simulink model "nonlinear_LQG"  (R2021b)
settings: Solver=VariableStepAuto  StartTime=0.0  StopTime=100  RelTol=1e-3
undefined symbols (not defined in the file): C1, K, sysKF
settings Model: Creator=Anubhav Paras  LastModifiedBy=vanshika
settings SolverCC: AlgebraicLoopSolver=TrustRegion
settings DebuggingCC: SFMachineParentedDataDiag=warning

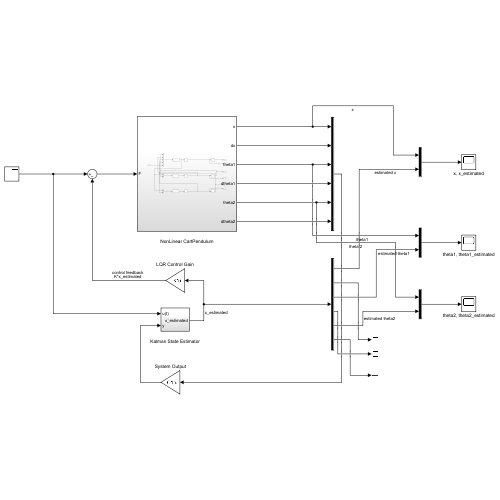
[thumbnail: Simulink's stored preview of the top-level diagram]
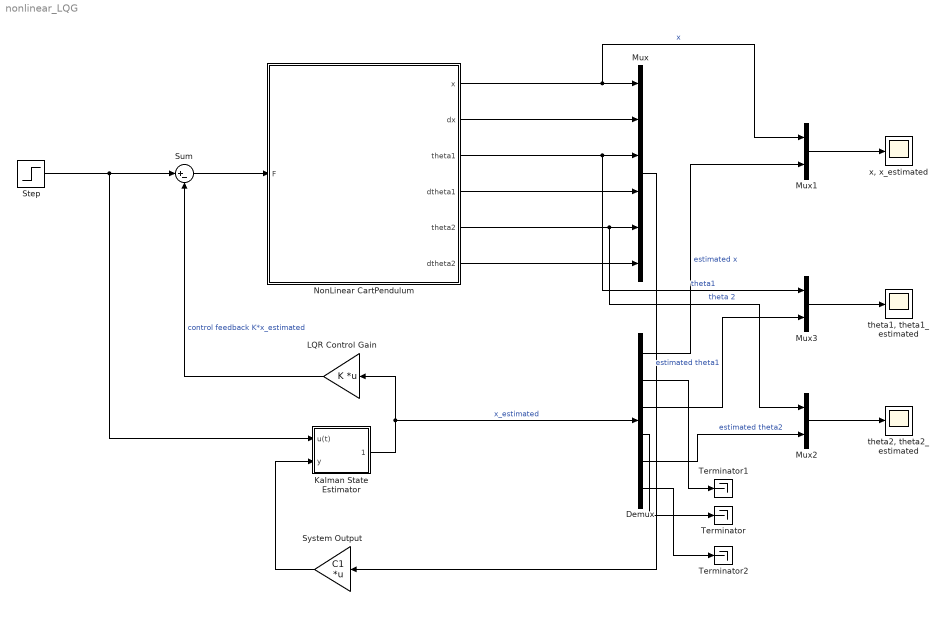
== system nonlinear_LQG ==
  " Kalman State Estimator" : Subsystem
  " NonLinear CartPendulum" : Subsystem
  Demux : Demux  Outputs=6
  LQR Control Gain : Gain  Gain=K  Multiplication=Matrix(K*u)
  Mux : Mux  Inputs=6
  Mux1 : Mux  Inputs=2
  Mux2 : Mux  Inputs=2
  Mux3 : Mux  Inputs=2
  Step : Step  SampleTime=5
  Sum : Sum  Inputs=|+-
  System Output : Gain  Gain=C1  Multiplication=Matrix(K*u)
  Terminator : Terminator
  Terminator1 : Terminator
  Terminator2 : Terminator
  "theta1, theta1_estimated" : Scope
  "theta2, theta2_estimated" : Scope
  "x, x_estimated" : Scope
  wires:
  System Output/1 -> " Kalman State Estimator"/2(y)
  " NonLinear CartPendulum"/1(x) -> Mux1/1, Mux/1  "x"
  Mux3/1 -> "theta1, theta1_estimated"/1
  Demux/1 -> Mux1/2  "estimated x"
  Mux2/1 -> "theta2, theta2_estimated"/1
  " Kalman State Estimator"/1(x_estimated) -> LQR Control Gain/1, Demux/1  "x_estimated"
  Demux/2 -> Terminator1/1
  Demux/4 -> Terminator/1
  Step/1 -> Sum/1, " Kalman State Estimator"/1(u(t))
  " NonLinear CartPendulum"/5(theta2) -> Mux2/1, Mux/5  "theta 2"
  " NonLinear CartPendulum"/2(dx) -> Mux/2
  Demux/5 -> Mux2/2  "estimated theta2"
  Mux1/1 -> "x, x_estimated"/1
  " NonLinear CartPendulum"/6(dtheta2) -> Mux/6
  Mux/1 -> System Output/1
  " NonLinear CartPendulum"/4(dtheta1) -> Mux/4
  Demux/6 -> Terminator2/1
  Demux/3 -> Mux3/2  "estimated theta1"
  " NonLinear CartPendulum"/3(theta1) -> Mux3/1, Mux/3  "theta1"
  Sum/1 -> " NonLinear CartPendulum"/1(F)
  LQR Control Gain/1 -> Sum/2  "control feedback K*x_estimated"

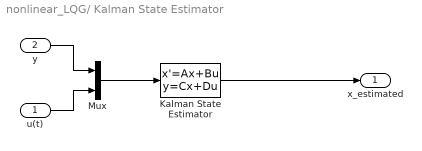
== system nonlinear_LQG/ Kalman State Estimator ==
  u(t) : Inport
  y : Inport  Port=2
  "Kalman State Estimator " : StateSpace  A=sysKF.a  B=sysKF.b  C=sysKF.c  D=sysKF.d  InitialCondition=0
  Mux : Mux  Inputs=2
  x_estimated : Outport
  wires:
  Mux/1 -> "Kalman State Estimator "/1
  "Kalman State Estimator "/1 -> x_estimated/1
  y/1 -> Mux/1
  u(t)/1 -> Mux/2

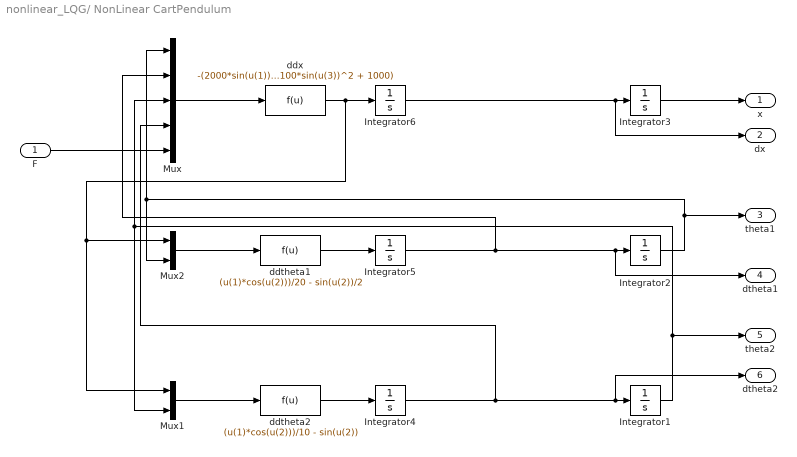
== system nonlinear_LQG/ NonLinear CartPendulum ==
  F : Inport
  Integrator1 : Integrator  InitialCondition=0.1
  Integrator2 : Integrator  InitialCondition=0.1
  Integrator3 : Integrator  InitialCondition=0.5
  Integrator4 : Integrator
  Integrator5 : Integrator
  Integrator6 : Integrator
  Mux : Mux  Inputs=5
  Mux1 : Mux  Inputs=2
  Mux2 : Mux  Inputs=2
  ddtheta1 : Fcn  Expr=(u(1)*cos(u(2)))/20 - sin(u(2))/2
  ddtheta2 : Fcn  Expr=(u(1)*cos(u(2)))/10 - sin(u(2))
  ddx : Fcn  Expr=-(2000*sin(u(1))*u(2)^2 + 1000*sin(u(3))*u(4)^2 - u(5) + 1000*cos(u(1))*sin(u(1)) - 1000*cos(u(3))*sin(u(3)))/(100*sin(u(1))^2 + 100*sin(u(3))^2 + 1000)
  x : Outport
  dx : Outport  Port=2
  theta1 : Outport  Port=3
  dtheta1 : Outport  Port=4
  theta2 : Outport  Port=5
  dtheta2 : Outport  Port=6
  wires:
  ddtheta2/1 -> Integrator4/1
  ddx/1 -> Mux1/1, Mux2/1, Integrator6/1
  Integrator6/1 -> dx/1, Integrator3/1
  Mux1/1 -> ddtheta2/1
  Integrator5/1 -> Mux/2, dtheta1/1, Integrator2/1
  Mux/1 -> ddx/1
  Integrator1/1 -> theta2/1, Mux1/2, Mux/3
  Integrator2/1 -> theta1/1, Mux2/2, Mux/1
  ddtheta1/1 -> Integrator5/1
  Integrator4/1 -> Mux/4, dtheta2/1, Integrator1/1
  Mux2/1 -> ddtheta1/1
  Integrator3/1 -> x/1
  F/1 -> Mux/5
